simulink model "glucose_subsystem"  (R2019a)
settings: Solver=VariableStepAuto  StartTime=0.0  StopTime=30.0  RelTol=1e-3
undefined symbols (not defined in the file): GLC_B, GPT_B, ILC_B, IPT_B, r_bHGP, r_bHGU
settings Model: Creator=rache  LastModifiedBy=rache
settings DataIOCC: ReturnWorkspaceOutputs=off
settings DebuggingCC: ArithmeticOperatorsInVariantConditions=warning

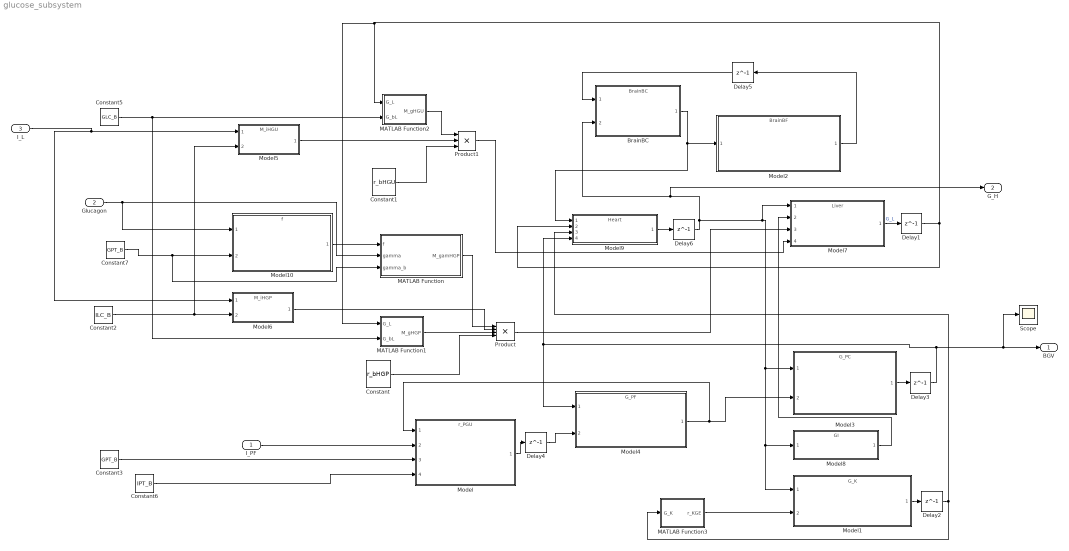
== system glucose_subsystem ==
  I_PF : Inport  OutMin=0
  Glucagon : Inport  Port=2
  I_L : Inport  Port=3
  BrainBC : ModelReference  ModelNameDialog=BrainBC  SimulationMode=Normal  ModelReferenceVersion=1.3
  Constant : Constant  Value=r_bHGP
  Constant1 : Constant  Value=r_bHGU
  Constant2 : Constant  Value=ILC_B
  Constant3 : Constant  Value=GPT_B
  Constant5 : Constant  Value=GLC_B
  Constant6 : Constant  Value=IPT_B
  Constant7 : Constant  Value=GPT_B
  Delay{1..6} (6 alike) : Delay  DelayLength=1  InitialCondition=0
  MATLAB Function : MATLAB Function  TreatAsAtomicUnit=on
  MATLAB Function1 : MATLAB Function  TreatAsAtomicUnit=on
  MATLAB Function2 : MATLAB Function  TreatAsAtomicUnit=on
  MATLAB Function3 : MATLAB Function  TreatAsAtomicUnit=on
  Model : ModelReference  ModelNameDialog=r_PGU  SimulationMode=Normal  ModelReferenceVersion=1.4
  Model1 : ModelReference  ModelNameDialog=G_K  SimulationMode=Normal  ModelReferenceVersion=1.1
  Model10 : ModelReference  ModelNameDialog=f  SimulationMode=Normal  ModelReferenceVersion=1.1
  Model2 : ModelReference  ModelNameDialog=BrainBF  SimulationMode=Normal  ModelReferenceVersion=1.3
  Model3 : ModelReference  ModelNameDialog=G_PC  SimulationMode=Normal  ModelReferenceVersion=1.2
  Model4 : ModelReference  ModelNameDialog=G_PF  SimulationMode=Normal  ModelReferenceVersion=1.1
  Model5 : ModelReference  ModelNameDialog=M_iHGU  SimulationMode=Normal  ModelReferenceVersion=1.2
  Model6 : ModelReference  ModelNameDialog=M_iHGP  SimulationMode=Normal  ModelReferenceVersion=1.1
  Model7 : ModelReference  ModelNameDialog=Liver  SimulationMode=Normal  ModelReferenceVersion=1.3
  Model8 : ModelReference  ModelNameDialog=GI  SimulationMode=Normal  ModelReferenceVersion=1.2
  Model9 : ModelReference  ModelNameDialog=Heart  SimulationMode=Normal  ModelReferenceVersion=1.2
  Product : Product  Inputs=4
  Product1 : Product  Inputs=3
  Scope : Scope
  BGV : Outport  OutMin=0
  G_H : Outport  Port=2  OutMin=0
  wires:
  Model7/1 -> Delay1/1  "G_L"
  Model/1 -> Delay4/1
  I_PF/1 -> Model/2
  Model10/1 -> MATLAB Function/1(f)
  MATLAB Function/1(M_gamHGP) -> Product/1
  Model6/1 -> Product/2
  MATLAB Function1/1(M_gHGP) -> Product/3
  Constant/1 -> Product/4
  Product/1 -> Model7/3
  MATLAB Function2/1(M_gHGU) -> Product1/1
  Model5/1 -> Product1/2
  Constant1/1 -> Product1/3
  MATLAB Function3/1(r_KGE) -> Model1/2
  Model4/1 -> Model/1, Model3/2
  Model3/1 -> Delay3/1
  Model8/1 -> Model7/2
  Model2/1 -> Delay5/1
  Model1/1 -> Delay2/1
  Product1/1 -> Model7/4
  BrainBC/1 -> Model9/1, Model2/1
  Model9/1 -> Delay6/1
  Delay1/1 -> MATLAB Function2/1(G_L), MATLAB Function1/1(G_L), Model9/2
  Delay2/1 -> Model9/3, MATLAB Function3/1(G_K)
  Delay3/1 -> Model4/1, Model9/4, Scope/1, BGV/1
  Delay4/1 -> Model4/2
  Delay5/1 -> BrainBC/1
  Delay6/1 -> G_H/1, BrainBC/2, Model1/1, Model8/1, Model3/1, Model7/1
  Constant3/1 -> Model/3
  Constant5/1 -> MATLAB Function1/2(G_bL), MATLAB Function2/2(G_bL)
  Constant2/1 -> Model5/2, Model6/2
  Constant6/1 -> Model/4
  Constant7/1 -> MATLAB Function/3(gamma_b), Model10/2
  Glucagon/1 -> Model10/1, MATLAB Function/2(gamma)
  I_L/1 -> Model5/1, Model6/1

== matlab function glucose_subsystem/MATLAB Function1 ==
  data: G_L input; M_gHGP output; G_bL input
function M_gHGP = fcn(G_L, G_bL)

M_gHGP = 1.42 - 1.41*tanh(0.62*(G_L/G_bL - 0.497));

== matlab function glucose_subsystem/MATLAB Function ==
  data: f input; M_gamHGP output; gamma input; gamma_b input
function M_gamHGP = fcn(f, gamma, gamma_b)

M_gamHGP = 2.7*tanh(0.39*gamma/gamma_b) - f;

== matlab function glucose_subsystem/MATLAB Function2 ==
  data: G_L input; M_gHGU output; G_bL input
function M_gHGU = fcn(G_L, G_bL)

M_gHGU = 5.66*(1 + tanh(2.44*(G_L/G_bL - 1.48)));

== matlab function glucose_subsystem/MATLAB Function3 ==
  data: G_K input; r_KGE output
function r_KGE = fcn(G_K)

r_KGE = 71+71*tanh(0.11*(G_K - 460));
